simulink model "fix_test"  (R2016a)
settings: Solver=VariableStepAuto  StartTime=0.0  StopTime=10e-6  RelTol=1e-3
values from neighbouring files (symbols this model uses):
  a = 4.7848e8    (= 478480000)    [DPLL_2ndType_2ndOrder.m]
  b = 1.7776e-4    (= 0.00017776)    [DPLL_2ndType_2ndOrder.m]
  c = 2.167e7    (= 21670000)    [DPLL_2ndType_2ndOrder.m]
  d = 1.735e-3    (= 0.001735)    [DPLL_2ndType_2ndOrder.m]
undefined symbols (not defined in the file): f0
settings Model: Creator=xzhang  LastModifiedBy=xzhang
settings SolverCC: ZeroCrossAlgorithm=Adaptive

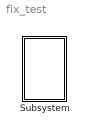
== system fix_test ==
  Subsystem : Subsystem

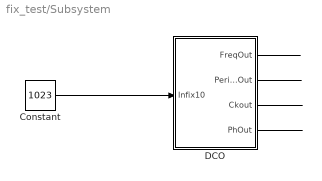
== system fix_test/Subsystem ==
  Constant : Constant  Value=1023  OutDataTypeStr=fixdt(0,10,0)
  DCO : Subsystem  mask{f0=f0, a=a, b=b, c=c, d=d}
      mask prompts: f0 "Free Running Freq.(Hz)"
  wires:
  Constant/1 -> DCO/1(Infix10)
  DCO/4(PhOut) -> ?
  DCO/3(Ckout) -> ?
  DCO/2(PeriodOut) -> ?
  DCO/1(FreqOut) -> ?

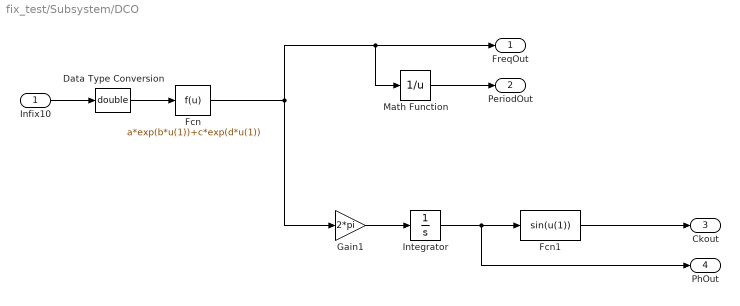
== system fix_test/Subsystem/DCO ==
  Infix10 : Inport  OutDataTypeStr=fixdt(0,10,0)
  Data Type Conversion : DataTypeConversion  OutDataTypeStr=double
  Fcn : Fcn  Expr=a*exp(b*u(1))+c*exp(d*u(1))
  Fcn1 : Fcn  Expr=sin(u(1))
  Gain1 : Gain  Gain=2*pi
  Integrator : Integrator
  Math Function : Math  Operator=reciprocal  SaturateOnIntegerOverflow=on
  FreqOut : Outport
  PeriodOut : Outport  Port=2
  Ckout : Outport  Port=3
  PhOut : Outport  Port=4
  wires:
  Fcn/1 -> FreqOut/1, Math Function/1, Gain1/1
  Fcn1/1 -> Ckout/1
  Integrator/1 -> PhOut/1, Fcn1/1
  Math Function/1 -> PeriodOut/1
  Infix10/1 -> Data Type Conversion/1
  Data Type Conversion/1 -> Fcn/1
  Gain1/1 -> Integrator/1
